simulink model "sim_sys_puma"  (R2017a)
settings: Solver=VariableStepAuto  StartTime=0.0  StopTime=3.2  MaxStep=0.01  RelTol=1e-4  EnableMultiTasking=on
values from neighbouring files (symbols this model uses):
  n_juncoes = size(vars, 1)    [animation.m]    (also in puma.m = 4; scara.m = 4)
undefined symbols (not defined in the file or in its folder): Q0
libraries: simulink x2
settings Model: Creator=julio  LastModifiedBy=julio
settings DataIOCC: LimitDataPoints=on  SaveOutput=off  SaveTime=off
settings OptimizationCC: ExpressionDepthLimit=2147483647  LifeSpan=1
settings DebuggingCC: AlgebraicLoopMsg=none  UnderspecifiedInitializationDetection=Classic  MergeDetectMultiDrivingBlocksExec=none  FcnCallInpInsideContextMsg=warning  AllowSymbolicDim=off  StateNameClashWarn=warning  SFUnexpectedBacktrackingDiag=warning  SFNoUnconditionalDefaultTransitionDiag=warning  SFExecutionAtInitializationDiag=none
settings GRTTargetCC: TargetLangStandard=C89/C90 (ANSI)  GeneratePreprocessorConditionals=Disable all  CombineOutputUpdateFcns=off  GRTInterface=on

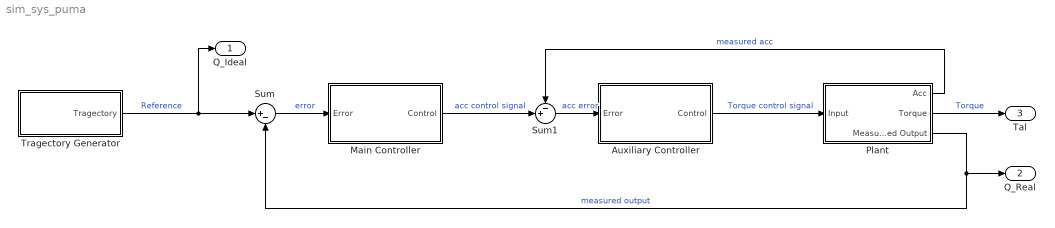
== system sim_sys_puma ==
  Auxiliary Controller : Subsystem
  Main Controller : Subsystem
  Plant : Subsystem
  Sum : Sum  Inputs=|+-
  Sum1 : Sum  Inputs=-+|
  Tragectory Generator : Subsystem
  Q_Ideal : Outport
  Q_Real : Outport  Port=2
  Tal : Outport  Port=3
  wires:
  Plant/1(Acc) -> Sum1/1  "measured acc"
  Main Controller/1(Control) -> Sum1/2  "acc control signal"
  Sum/1 -> Main Controller/1(Error)  "error"
  Tragectory Generator/1(Tragectory) -> Q_Ideal/1, Sum/1  "Reference"
  Plant/2(Torque) -> Tal/1  "Torque"
  Plant/3(Measured Output) -> Q_Real/1, Sum/2  "measured output"
  Auxiliary Controller/1(Control) -> Plant/1(Input)  "Torque control signal"
  Sum1/1 -> Auxiliary Controller/1(Error)  "acc error"

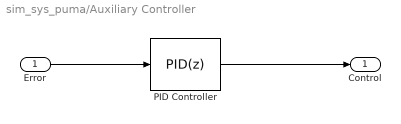
== system sim_sys_puma/Auxiliary Controller ==
  Error : Inport  PortDimensions=n_juncoes
  PID Controller : simulink/Continuous/PID Controller  Controller=PID  TimeDomain=Discrete-time  SampleTime=0.001  IntegratorMethod=Forward Euler  FilterMethod=Forward Euler  Form=Ideal  UseFilter=off  ControllerParametersSource=internal  P=8  I=12  D=10  N=20  InitialConditionSource=internal  InitialConditionForIntegrator=0  InitialConditionForFilter=0  ExternalReset=none  LimitOutput=off  UpperSaturationLimit=inf  LowerSaturationLimit=-inf  LinearizeAsGain=on  AntiWindupMode=none  Kb=1  TrackingMode=off  Kt=1  PParamMin=[]  PParamMax=[]  IParamMin=[]  IParamMax=[]  DParamMin=[]  DParamMax=[]  NParamMin=[]  NParamMax=[]  KbParamMin=[]  KbParamMax=[]  KtParamMin=[]  KtParamMax=[]  POutMin=[]  POutMax=[]  IOutMin=[]  IOutMax=[]  DOutMin=[]  DOutMax=[]  NOutMin=[]  NOutMax=[]  KbOutMin=[]  KbOutMax=[]  KtOutMin=[]  KtOutMax=[]  IntegratorOutMin=[]  IntegratorOutMax=[]  FilterOutMin=[]  FilterOutMax=[]  SumOutMin=[]  SumOutMax=[]  SumI1OutMin=[]  SumI1OutMax=[]  SumI2OutMin=[]  SumI2OutMax=[]  SumI3OutMin=[]  SumI3OutMax=[]  SumDOutMin=[]  SumDOutMax=[]  SaturationOutMin=[]  SaturationOutMax=[]  IntegratorContinuousStateAttributes=''  IntegratorStateMustResolveToSignalObject=off  IntegratorRTWStateStorageClass=Auto  FilterContinuousStateAttributes=''  FilterStateMustResolveToSignalObject=off  FilterRTWStateStorageClass=Auto  DifferentiatorICPrevScaledInput=0  DifferentiatorOutMin=[]  DifferentiatorOutMax=[]  InitialConditionSetting=State (most efficient)
  Control : Outport  PortDimensions=n_juncoes
  wires:
  Error/1 -> PID Controller/1
  PID Controller/1 -> Control/1

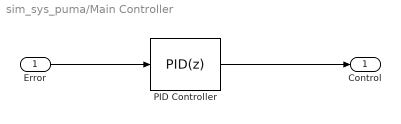
== system sim_sys_puma/Main Controller ==
  Error : Inport  PortDimensions=n_juncoes
  PID Controller : simulink/Continuous/PID Controller  Controller=PID  TimeDomain=Discrete-time  SampleTime=0.005  IntegratorMethod=Forward Euler  FilterMethod=Forward Euler  Form=Ideal  UseFilter=off  ControllerParametersSource=internal  P=8  I=5  D=10  N=20  InitialConditionSource=internal  InitialConditionForIntegrator=0  InitialConditionForFilter=0  ExternalReset=none  LimitOutput=off  UpperSaturationLimit=inf  LowerSaturationLimit=-inf  LinearizeAsGain=on  AntiWindupMode=none  Kb=1  TrackingMode=off  Kt=1  PParamMin=[]  PParamMax=[]  IParamMin=[]  IParamMax=[]  DParamMin=[]  DParamMax=[]  NParamMin=[]  NParamMax=[]  KbParamMin=[]  KbParamMax=[]  KtParamMin=[]  KtParamMax=[]  POutMin=[]  POutMax=[]  IOutMin=[]  IOutMax=[]  DOutMin=[]  DOutMax=[]  NOutMin=[]  NOutMax=[]  KbOutMin=[]  KbOutMax=[]  KtOutMin=[]  KtOutMax=[]  IntegratorOutMin=[]  IntegratorOutMax=[]  FilterOutMin=[]  FilterOutMax=[]  SumOutMin=[]  SumOutMax=[]  SumI1OutMin=[]  SumI1OutMax=[]  SumI2OutMin=[]  SumI2OutMax=[]  SumI3OutMin=[]  SumI3OutMax=[]  SumDOutMin=[]  SumDOutMax=[]  SaturationOutMin=[]  SaturationOutMax=[]  IntegratorContinuousStateAttributes=''  IntegratorStateMustResolveToSignalObject=off  IntegratorRTWStateStorageClass=Auto  FilterContinuousStateAttributes=''  FilterStateMustResolveToSignalObject=off  FilterRTWStateStorageClass=Auto  DifferentiatorICPrevScaledInput=0  DifferentiatorOutMin=[]  DifferentiatorOutMax=[]  InitialConditionSetting=State (most efficient)
  Control : Outport  PortDimensions=n_juncoes
  wires:
  Error/1 -> PID Controller/1
  PID Controller/1 -> Control/1

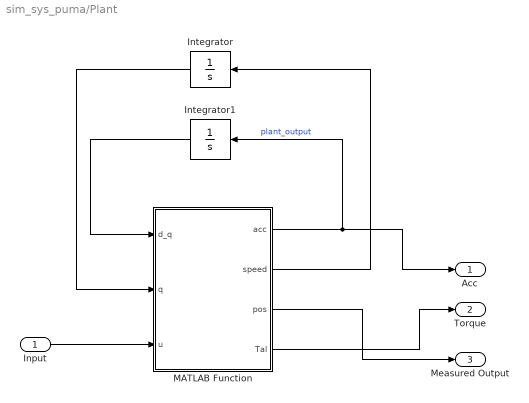
== system sim_sys_puma/Plant ==
  Input : Inport  PortDimensions=n_juncoes
  Integrator : Integrator  InitialCondition=Q0
  Integrator1 : Integrator  InitialCondition=zeros(n_juncoes, 1)
  MATLAB Function : MATLAB Function  TreatAsAtomicUnit=on
  Acc : Outport
  Torque : Outport  Port=2  PortDimensions=n_juncoes
  Measured Output : Outport  Port=3  PortDimensions=n_juncoes
  wires:
  Input/1 -> MATLAB Function/3(u)
  MATLAB Function/2(speed) -> Integrator/1
  MATLAB Function/1(acc) -> Acc/1, Integrator1/1  "plant_output"
  MATLAB Function/3(pos) -> Measured Output/1
  Integrator/1 -> MATLAB Function/2(q)
  Integrator1/1 -> MATLAB Function/1(d_q)
  MATLAB Function/4(Tal) -> Torque/1

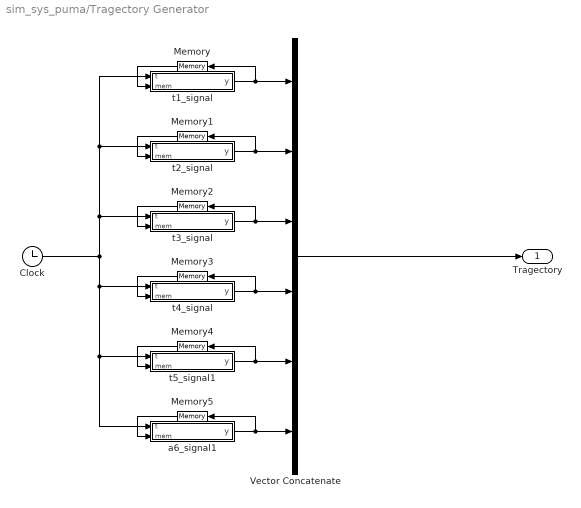
== system sim_sys_puma/Tragectory Generator ==
  Clock : Clock
  Memory : Memory  X0=Q0(1)
  Memory1 : Memory  X0=Q0(2)
  Memory2 : Memory  X0=Q0(3)
  Memory3 : Memory  X0=Q0(4)
  Memory4 : Memory  X0=Q0(3)
  Memory5 : Memory  X0=Q0(4)
  Vector Concatenate : Concatenate  NumInputs=6
  a6_signal1 : MATLAB Function  TreatAsAtomicUnit=on
  t1_signal : MATLAB Function  TreatAsAtomicUnit=on
  t2_signal : MATLAB Function  TreatAsAtomicUnit=on
  t3_signal : MATLAB Function  TreatAsAtomicUnit=on
  t4_signal : MATLAB Function  TreatAsAtomicUnit=on
  t5_signal1 : MATLAB Function  TreatAsAtomicUnit=on
  Tragectory : Outport
  wires:
  Vector Concatenate/1 -> Tragectory/1
  t2_signal/1(y) -> Vector Concatenate/2, Memory1/1
  Memory1/1 -> t2_signal/2(mem)
  Memory/1 -> t1_signal/2(mem)
  t1_signal/1(y) -> Memory/1, Vector Concatenate/1
  t4_signal/1(y) -> Vector Concatenate/4, Memory3/1
  t3_signal/1(y) -> Vector Concatenate/3, Memory2/1
  Memory3/1 -> t4_signal/2(mem)
  Memory2/1 -> t3_signal/2(mem)
  Memory4/1 -> t5_signal1/2(mem)
  a6_signal1/1(y) -> Vector Concatenate/6, Memory5/1
  t5_signal1/1(y) -> Vector Concatenate/5, Memory4/1
  Memory5/1 -> a6_signal1/2(mem)
  Clock/1 -> t2_signal/1(t), t1_signal/1(t), t3_signal/1(t), a6_signal1/1(t), t5_signal1/1(t), t4_signal/1(t)

== matlab function sim_sys_puma/Tragectory Generator/t5_signal1 ==
  data: t input; y output; mem input
function y = fcn(t,mem)
    
    tempos = [
        [     0,     1]
        [ 11/10, 21/10]
        [  11/5,  16/5]
    ];

    period = max(max(tempos));
    t = mod(t,period);
    
    c = [
        [ 0, 0, 0, 0, 0, 0]
        [ 0, 0, 0, 0, 0, 0]
        [ 0, 0, 0, 0, 0, 0]
    ];

    i = 0;
    
    for j=1:size(tempos,1)
        if(t >= tempos(j,1))
            if t<= tempos(j,2)
                i = j;
                break;
            end
        end
    end
    
    if i> 0
        y = c(i,1) + c(i,2)*t + c(i,3)*t^2 + c(i,4)*t^3 + c(i,5)*t^4 + c(i,6)*t^5;
    else
        y = mem;
    end
    
end

== matlab function sim_sys_puma/Plant/MATLAB Function ==
  data: d_q input; acc output; q input; speed output; u input size=n_juncoes; pos output; Tal output
function [acc, speed, pos, Tal] = system(d_q, q, u)

    t1 = q(1);
    t2 = q(2);
    t3 = q(3);
    t4 = q(4);
    t5 = q(5);
    a6 = q(6);
    w1 = d_q(1);
    w2 = d_q(2);
    w3 = d_q(3);
    w4 = d_q(4);
    w5 = d_q(5);
    w6 = d_q(6);
    
    D = [
        [  (93*sin(t3 + t4 + t5))/2500 + (96*sin(t3 + t4))/125 + (36*cos(t3))/25 + (32*sin(t3 + t4)^2)/25 + (12*cos(t3)^2)/5 + (31*sin(t3 + t4 + t5)*sin(t3 + t4))/250 + (31*sin(t3 + t4 + t5)*cos(t3))/250 + (459*sin(t3 + t4 + t5)^2)/20000 + (64*sin(t3 + t4)*cos(t3))/25 + 917/1250, (93*sin(t3 + t4 + t5))/2500 + (96*sin(t3 + t4))/125 + (36*cos(t3))/25 + (32*sin(t3 + t4)^2)/25 + (12*cos(t3)^2)/5 + (31*sin(t3 + t4 + t5)*sin(t3 + t4))/250 + (31*sin(t3 + t4 + t5)*cos(t3))/250 + (459*sin(t3 + t4 + t5)^2)/20000 + (64*sin(t3 + t4)*cos(t3))/25 + 1459/2500,                                                                        0,                                                                        0,                                                     0,                                         0]
        [ (93*sin(t3 + t4 + t5))/2500 + (96*sin(t3 + t4))/125 + (36*cos(t3))/25 + (32*sin(t3 + t4)^2)/25 + (12*cos(t3)^2)/5 + (31*sin(t3 + t4 + t5)*sin(t3 + t4))/250 + (31*sin(t3 + t4 + t5)*cos(t3))/250 + (459*sin(t3 + t4 + t5)^2)/20000 + (64*sin(t3 + t4)*cos(t3))/25 + 1459/2500, (93*sin(t3 + t4 + t5))/2500 + (96*sin(t3 + t4))/125 + (36*cos(t3))/25 + (32*sin(t3 + t4)^2)/25 + (12*cos(t3)^2)/5 + (31*sin(t3 + t4 + t5)*sin(t3 + t4))/250 + (31*sin(t3 + t4 + t5)*cos(t3))/250 + (459*sin(t3 + t4 + t5)^2)/20000 + (64*sin(t3 + t4)*cos(t3))/25 + 1459/2500,                                                                        0,                                                                        0,                                                     0,                                         0]
        [                                                                                                                                                                                                                                                                             0,                                                                                                                                                                                                                                                                             0, (31*sin(t4 + t5))/250 + (31*cos(t5))/250 + (64*sin(t4))/25 + 79259/20000, (31*sin(t4 + t5))/500 + (31*cos(t5))/250 + (32*sin(t4))/25 + 29259/20000, (31*sin(t4 + t5))/500 + (31*cos(t5))/500 + 1659/20000, sin(t4 + t5)/100 + cos(t5)/100 + 183/8000]
        [                                                                                                                                                                                                                                                                             0,                                                                                                                                                                                                                                                                             0, (31*sin(t4 + t5))/500 + (31*cos(t5))/250 + (32*sin(t4))/25 + 29259/20000,                                           (31*cos(t5))/250 + 29259/20000,                         (31*cos(t5))/500 + 1659/20000,                    cos(t5)/100 + 183/8000]
        [                                                                                                                                                                                                                                                                             0,                                                                                                                                                                                                                                                                             0,                    (31*sin(t4 + t5))/500 + (31*cos(t5))/500 + 1659/20000,                                            (31*cos(t5))/500 + 1659/20000,                                            1659/20000,                                  183/8000]
        [                                                                                                                                                                                                                                                                             0,                                                                                                                                                                                                                                                                             0,                                sin(t4 + t5)/100 + cos(t5)/100 + 183/8000,                                                   cos(t5)/100 + 183/8000,                                              183/8000,                                    17/800]
    ];

    C = [
        [ (459*w3*sin(2*t3 + 2*t4 + 2*t5))/40000 - (6*w3*sin(2*t3))/5 + (459*w4*sin(2*t3 + 2*t4 + 2*t5))/40000 + (459*w5*sin(2*t3 + 2*t4 + 2*t5))/40000 + (16*w3*sin(2*t3 + 2*t4))/25 + (16*w4*sin(2*t3 + 2*t4))/25 + (31*w3*cos(2*t3 + t4 + t5))/500 + (31*w4*cos(2*t3 + t4 + t5))/1000 + (31*w5*cos(2*t3 + t4 + t5))/1000 + (48*w3*cos(t3 + t4))/125 + (48*w4*cos(t3 + t4))/125 + (31*w4*cos(t4 + t5))/1000 + (31*w5*cos(t4 + t5))/1000 + (16*w4*cos(t4))/25 - (18*w3*sin(t3))/25 - (31*w5*sin(t5))/1000 + (31*w3*sin(2*t3 + 2*t4 + t5))/500 + (31*w4*sin(2*t3 + 2*t4 + t5))/500 + (31*w5*sin(2*t3 + 2*t4 + t5))/1000 + (32*w3*cos(2*t3 + t4))/25 + (16*w4*cos(2*t3 + t4))/25 + (93*w3*cos(t3 + t4 + t5))/5000 + (93*w4*cos(t3 + t4 + t5))/5000 + (93*w5*cos(t3 + t4 + t5))/5000, (459*w3*sin(2*t3 + 2*t4 + 2*t5))/40000 - (6*w3*sin(2*t3))/5 + (459*w4*sin(2*t3 + 2*t4 + 2*t5))/40000 + (459*w5*sin(2*t3 + 2*t4 + 2*t5))/40000 + (16*w3*sin(2*t3 + 2*t4))/25 + (16*w4*sin(2*t3 + 2*t4))/25 + (31*w3*cos(2*t3 + t4 + t5))/500 + (31*w4*cos(2*t3 + t4 + t5))/1000 + (31*w5*cos(2*t3 + t4 + t5))/1000 + (48*w3*cos(t3 + t4))/125 + (48*w4*cos(t3 + t4))/125 + (31*w4*cos(t4 + t5))/1000 + (31*w5*cos(t4 + t5))/1000 + (16*w4*cos(t4))/25 - (18*w3*sin(t3))/25 - (31*w5*sin(t5))/1000 + (31*w3*sin(2*t3 + 2*t4 + t5))/500 + (31*w4*sin(2*t3 + 2*t4 + t5))/500 + (31*w5*sin(2*t3 + 2*t4 + t5))/1000 + (32*w3*cos(2*t3 + t4))/25 + (16*w4*cos(2*t3 + t4))/25 + (93*w3*cos(t3 + t4 + t5))/5000 + (93*w4*cos(t3 + t4 + t5))/5000 + (93*w5*cos(t3 + t4 + t5))/5000, ((w1 + w2)*(51200*cos(2*t3 + t4) + 744*cos(t3 + t4 + t5) - 48000*sin(2*t3) + 459*sin(2*t3 + 2*t4 + 2*t5) + 25600*sin(2*t3 + 2*t4) + 2480*cos(2*t3 + t4 + t5) + 15360*cos(t3 + t4) - 28800*sin(t3) + 2480*sin(2*t3 + 2*t4 + t5)))/40000, ((w1 + w2)*(25600*cos(2*t3 + t4) + 744*cos(t3 + t4 + t5) + 459*sin(2*t3 + 2*t4 + 2*t5) + 25600*sin(2*t3 + 2*t4) + 1240*cos(2*t3 + t4 + t5) + 15360*cos(t3 + t4) + 1240*cos(t4 + t5) + 25600*cos(t4) + 2480*sin(2*t3 + 2*t4 + t5)))/40000, (cos(t3 + t4 + t5)*(w1 + w2)*(459*sin(t3 + t4 + t5) + 1240*sin(t3 + t4) + 1240*cos(t3) + 372))/20000,                                                           0]
        [ (459*w3*sin(2*t3 + 2*t4 + 2*t5))/40000 - (6*w3*sin(2*t3))/5 + (459*w4*sin(2*t3 + 2*t4 + 2*t5))/40000 + (459*w5*sin(2*t3 + 2*t4 + 2*t5))/40000 + (16*w3*sin(2*t3 + 2*t4))/25 + (16*w4*sin(2*t3 + 2*t4))/25 + (31*w3*cos(2*t3 + t4 + t5))/500 + (31*w4*cos(2*t3 + t4 + t5))/1000 + (31*w5*cos(2*t3 + t4 + t5))/1000 + (48*w3*cos(t3 + t4))/125 + (48*w4*cos(t3 + t4))/125 + (31*w4*cos(t4 + t5))/1000 + (31*w5*cos(t4 + t5))/1000 + (16*w4*cos(t4))/25 - (18*w3*sin(t3))/25 - (31*w5*sin(t5))/1000 + (31*w3*sin(2*t3 + 2*t4 + t5))/500 + (31*w4*sin(2*t3 + 2*t4 + t5))/500 + (31*w5*sin(2*t3 + 2*t4 + t5))/1000 + (32*w3*cos(2*t3 + t4))/25 + (16*w4*cos(2*t3 + t4))/25 + (93*w3*cos(t3 + t4 + t5))/5000 + (93*w4*cos(t3 + t4 + t5))/5000 + (93*w5*cos(t3 + t4 + t5))/5000, (459*w3*sin(2*t3 + 2*t4 + 2*t5))/40000 - (6*w3*sin(2*t3))/5 + (459*w4*sin(2*t3 + 2*t4 + 2*t5))/40000 + (459*w5*sin(2*t3 + 2*t4 + 2*t5))/40000 + (16*w3*sin(2*t3 + 2*t4))/25 + (16*w4*sin(2*t3 + 2*t4))/25 + (31*w3*cos(2*t3 + t4 + t5))/500 + (31*w4*cos(2*t3 + t4 + t5))/1000 + (31*w5*cos(2*t3 + t4 + t5))/1000 + (48*w3*cos(t3 + t4))/125 + (48*w4*cos(t3 + t4))/125 + (31*w4*cos(t4 + t5))/1000 + (31*w5*cos(t4 + t5))/1000 + (16*w4*cos(t4))/25 - (18*w3*sin(t3))/25 - (31*w5*sin(t5))/1000 + (31*w3*sin(2*t3 + 2*t4 + t5))/500 + (31*w4*sin(2*t3 + 2*t4 + t5))/500 + (31*w5*sin(2*t3 + 2*t4 + t5))/1000 + (32*w3*cos(2*t3 + t4))/25 + (16*w4*cos(2*t3 + t4))/25 + (93*w3*cos(t3 + t4 + t5))/5000 + (93*w4*cos(t3 + t4 + t5))/5000 + (93*w5*cos(t3 + t4 + t5))/5000, ((w1 + w2)*(51200*cos(2*t3 + t4) + 744*cos(t3 + t4 + t5) - 48000*sin(2*t3) + 459*sin(2*t3 + 2*t4 + 2*t5) + 25600*sin(2*t3 + 2*t4) + 2480*cos(2*t3 + t4 + t5) + 15360*cos(t3 + t4) - 28800*sin(t3) + 2480*sin(2*t3 + 2*t4 + t5)))/40000, ((w1 + w2)*(25600*cos(2*t3 + t4) + 744*cos(t3 + t4 + t5) + 459*sin(2*t3 + 2*t4 + 2*t5) + 25600*sin(2*t3 + 2*t4) + 1240*cos(2*t3 + t4 + t5) + 15360*cos(t3 + t4) + 1240*cos(t4 + t5) + 25600*cos(t4) + 2480*sin(2*t3 + 2*t4 + t5)))/40000, (cos(t3 + t4 + t5)*(w1 + w2)*(459*sin(t3 + t4 + t5) + 1240*sin(t3 + t4) + 1240*cos(t3) + 372))/20000,                                                           0]
        [                                                                                                                                                                                                                                                                                                                                                                                                                                                                                                                                  -((w1 + w2)*(51200*cos(2*t3 + t4) + 744*cos(t3 + t4 + t5) - 48000*sin(2*t3) + 459*sin(2*t3 + 2*t4 + 2*t5) + 25600*sin(2*t3 + 2*t4) + 2480*cos(2*t3 + t4 + t5) + 15360*cos(t3 + t4) - 28800*sin(t3) + 2480*sin(2*t3 + 2*t4 + t5)))/40000,                                                                                                                                                                                                                                                                                                                                                                                                                                                                                                                                  -((w1 + w2)*(51200*cos(2*t3 + t4) + 744*cos(t3 + t4 + t5) - 48000*sin(2*t3) + 459*sin(2*t3 + 2*t4 + 2*t5) + 25600*sin(2*t3 + 2*t4) + 2480*cos(2*t3 + t4 + t5) + 15360*cos(t3 + t4) - 28800*sin(t3) + 2480*sin(2*t3 + 2*t4 + t5)))/40000,                                                                                                                                           w4*((31*cos(t4 + t5))/500 + (32*cos(t4))/25) + w5*((31*cos(t4 + t5))/500 - (31*sin(t5))/500),                                                                      w3*((31*cos(t4 + t5))/500 + (32*cos(t4))/25) + w4*((31*cos(t4 + t5))/500 + (32*cos(t4))/25) + (w6*cos(t4 + t5))/200 + w5*((31*cos(t4 + t5))/500 - (31*sin(t5))/500),                                       ((cos(t4 + t5) - sin(t5))*(62*w3 + 62*w4 + 62*w5 + 5*w6))/1000, (w4*cos(t4 + t5))/200 + w5*(cos(t4 + t5)/200 - sin(t5)/200)]
        [                                                                                                                                                                                                                                                                                                                                                                                                                                                                                                                                -((w1 + w2)*(25600*cos(2*t3 + t4) + 744*cos(t3 + t4 + t5) + 459*sin(2*t3 + 2*t4 + 2*t5) + 25600*sin(2*t3 + 2*t4) + 1240*cos(2*t3 + t4 + t5) + 15360*cos(t3 + t4) + 1240*cos(t4 + t5) + 25600*cos(t4) + 2480*sin(2*t3 + 2*t4 + t5)))/40000,                                                                                                                                                                                                                                                                                                                                                                                                                                                                                                                                -((w1 + w2)*(25600*cos(2*t3 + t4) + 744*cos(t3 + t4 + t5) + 459*sin(2*t3 + 2*t4 + 2*t5) + 25600*sin(2*t3 + 2*t4) + 1240*cos(2*t3 + t4 + t5) + 15360*cos(t3 + t4) + 1240*cos(t4 + t5) + 25600*cos(t4) + 2480*sin(2*t3 + 2*t4 + t5)))/40000,                                                                                                                                           - w3*((31*cos(t4 + t5))/500 + (32*cos(t4))/25) - (w6*cos(t4 + t5))/200 - (31*w5*sin(t5))/500,                                                                                                                                                                                                                     -(31*w5*sin(t5))/500,                                                       -(sin(t5)*(62*w3 + 62*w4 + 62*w5 + 5*w6))/1000,                  - (w3*cos(t4 + t5))/200 - (w5*sin(t5))/200]
        [                                                                                                                                                                                                                                                                                                                                                                                                                                                                                                                                                                                                                                                                    -(cos(t3 + t4 + t5)*(w1 + w2)*(459*sin(t3 + t4 + t5) + 1240*sin(t3 + t4) + 1240*cos(t3) + 372))/20000,                                                                                                                                                                                                                                                                                                                                                                                                                                                                                                                                                                                                                                                                    -(cos(t3 + t4 + t5)*(w1 + w2)*(459*sin(t3 + t4 + t5) + 1240*sin(t3 + t4) + 1240*cos(t3) + 372))/20000,                                                                                                                              (31*w4*sin(t5))/500 - w3*((31*cos(t4 + t5))/500 - (31*sin(t5))/500) - w6*(cos(t4 + t5)/200 - sin(t5)/200),                                                                                                                                                                                                    (sin(t5)*(62*w3 + 62*w4 + 5*w6))/1000,                                                                                                    0,      (w4*sin(t5))/200 - w3*(cos(t4 + t5)/200 - sin(t5)/200)]
        [                                                                                                                                                                                                                                                                                                                                                                                                                                                                                                                                                                                                                                                                                                                                                                        0,                                                                                                                                                                                                                                                                                                                                                                                                                                                                                                                                                                                                                                                                                                                                                                        0,                                                                                                                                                                            (w4*cos(t4 + t5))/200 + w5*(cos(t4 + t5)/200 - sin(t5)/200),                                                                                                                                                                                                 (w3*cos(t4 + t5))/200 - (w5*sin(t5))/200,                                               w3*(cos(t4 + t5)/200 - sin(t5)/200) - (w4*sin(t5))/200,                                                           0]
    ];

    g = [
                                                                                       0
                                                                                       0
         - (30411*sin(t3 + t4 + t5))/20000 - (3924*sin(t3 + t4))/125 - (2943*cos(t3))/50
                             - (30411*sin(t3 + t4 + t5))/20000 - (3924*sin(t3 + t4))/125
                                                        -(30411*sin(t3 + t4 + t5))/20000
                                                                                       0
    ];

    acc = inv(D)*(u - C*d_q - g);
    Tal = D*acc + C*d_q + g;
    speed = d_q;
    pos = q;
end

== matlab function sim_sys_puma/Tragectory Generator/a6_signal1 ==
  data: t input; y output; mem input
function y = fcn(t,mem)
    
    tempos = [
        [     0,     1]
        [ 11/10, 21/10]
        [  11/5,  16/5]
    ];

    period = max(max(tempos));
    t = mod(t,period);
    
    c = [
        [ 0, 0, 0, 0, 0, 0]
        [ 0, 0, 0, 0, 0, 0]
        [ 0, 0, 0, 0, 0, 0]
    ];

    i = 0;
    
    for j=1:size(tempos,1)
        if(t >= tempos(j,1))
            if t<= tempos(j,2)
                i = j;
                break;
            end
        end
    end
    
    if i> 0
        y = c(i,1) + c(i,2)*t + c(i,3)*t^2 + c(i,4)*t^3 + c(i,5)*t^4 + c(i,6)*t^5;
    else
        y = mem;
    end
    
end

== matlab function sim_sys_puma/Tragectory Generator/t3_signal ==
  data: t input; y output; mem input
function y = fcn(t,mem)
    
    tempos = [
        [     0,     1]
        [ 11/10, 21/10]
        [  11/5,  16/5]
    ];

    period = max(max(tempos));
    t = mod(t,period);
    
    c = [
        [ 6643266975759255/4503599627370496,                                0,                                 0, -829151420652521/562949953421312,  2487454261957563/1125899906842624, -3979926819132101/4503599627370496]
[ -1232224976939381/562949953421312, 1763226510431021/140737488355328, -4885129725869491/281474976710656, 3273495117533395/281474976710656, -4229549546207341/1125899906842624, 8459099092414667/18014398509481984]
[    -875815913792995/4398046511104,   1709595497499089/4398046511104,   -2622674910936113/8796093022208,  3977429263077929/35184372088832,  -2980312398791057/140737488355328,  7064444204541785/4503599627370496]

    ];

    i = 0;
    
    for j=1:size(tempos,1)
        if(t >= tempos(j,1))
            if t<= tempos(j,2)
                i = j;
                break;
            end
        end
    end
    
    if i> 0
        y = c(i,1) + c(i,2)*t + c(i,3)*t^2 + c(i,4)*t^3 + c(i,5)*t^4 + c(i,6)*t^5;
    else
        y = mem;
    end
    
end

== matlab function sim_sys_puma/Tragectory Generator/t1_signal ==
  data: t input; y output; mem input
function y = fcn(t, mem)
    
    tempos = [
        [     0,     1]
        [ 11/10, 21/10]
        [  11/5,  16/5]
    ];

    period = max(max(tempos));
    t = mod(t,period);
    
    c = [
        [ -884279719006747/562949953421312,                              0,                               0, 6084582650169709/1125899906842624, -2281718493813641/281474976710656,  7301499180203651/2251799813685248]
[  1672547114383301/35184372088832, -760967378419923/4398046511104,   527076972065747/2199023255552,   -1412764034072329/8796093022208,   3650749590065771/70368744177664, -7301499180131529/1125899906842624]
[  -1832477936985719/4398046511104,  883481400797525/1099511627776, -1355340785314389/2199023255552,    1027724038246955/4398046511104,  -3080319966623631/70368744177664,  7301499180144925/2251799813685248]
    ];

    i = 0;
    
    for j=1:size(tempos,1)
        if(t >= tempos(j,1))
            if t<= tempos(j,2)
                i = j;
                break;
            end
        end
    end
    
    if i> 0
        y = c(i,1) + c(i,2)*t + c(i,3)*t^2 + c(i,4)*t^3 + c(i,5)*t^4 + c(i,6)*t^5;
    else
        y = mem;
    end
    
end

== matlab function sim_sys_puma/Tragectory Generator/t2_signal ==
  data: t input; y output; mem input
function y = fcn(t,mem)
    
    tempos = [
        [     0,     1]
        [ 11/10, 21/10]
        [  11/5,  16/5]
    ];

    period = max(max(tempos));
    t = mod(t,period);
    
    c = [
        [ 811458320100571/281474976710656,                                 0,                                0, -6451440309747949/4503599627370496, 4838580232310961/2251799813685248,  -3870864185848769/4503599627370496]
[ 815202598799567/140737488355328, -1530606508498259/140737488355328, 2120320704413171/140737488355328,  -1420813747636169/140737488355328,   458943875414105/140737488355328, -7343102006625667/18014398509481984]
[  -145887965392515/2199023255552,     588329929643059/4398046511104, -1805103193223029/17592186044416,   5475074500207915/140737488355328, -1025626814331273/140737488355328,   4862230823496419/9007199254740992]

    ];

    i = 0;
    
    for j=1:size(tempos,1)
        if(t >= tempos(j,1))
            if t<= tempos(j,2)
                i = j;
                break;
            end
        end
    end
    
    if i> 0
        y = c(i,1) + c(i,2)*t + c(i,3)*t^2 + c(i,4)*t^3 + c(i,5)*t^4 + c(i,6)*t^5;
    else
        y = mem;
    end
    
end

== matlab function sim_sys_puma/Tragectory Generator/t4_signal ==
  data: t input; y output; mem input
function y = fcn(t,mem)
    
    tempos = [
        [     0,     1]
        [ 11/10, 21/10]
        [  11/5,  16/5]
    ];

    period = max(max(tempos));
    t = mod(t,period);
    
    c = [
        [ -6021299811766973/2251799813685248,                                 0,                                  0,  1121232153837545/140737488355328,  -6727392923025269/562949953421312,  5381914338420215/1125899906842624]
[  -1324250185646977/562949953421312, 3810794255491753/2251799813685248, -5279022345269959/2251799813685248, 1768720058863445/1125899906842624, -4570582117116837/9007199254740992, 4570582117116829/72057594037927936]
[      671406822247817/1099511627776,   -2610755442457407/2199023255552,     4005136190133533/4398046511104,   -3037003522400647/8796093022208,    2275645562575885/35184372088832,  -2697061407497353/562949953421312]

    ];

    i = 0;
    
    for j=1:size(tempos,1)
        if(t >= tempos(j,1))
            if t<= tempos(j,2)
                i = j;
                break;
            end
        end
    end
    
    if i> 0
        y = c(i,1) + c(i,2)*t + c(i,3)*t^2 + c(i,4)*t^3 + c(i,5)*t^4 + c(i,6)*t^5;
    else
        y = mem;
    end
    
end
